simulink library "INT_CoTS_MechDem"  (R2016b)
settings: Solver=VariableStepAuto  StartTime=0.0  StopTime=10.0  RelTol=1e-3
settings Model: Creator=xinchangran  LastModifiedBy=xinchangran

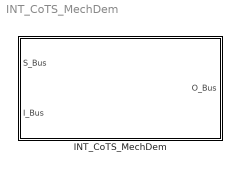
== system INT_CoTS_MechDem ==
  INT_CoTS_MechDem : Subsystem

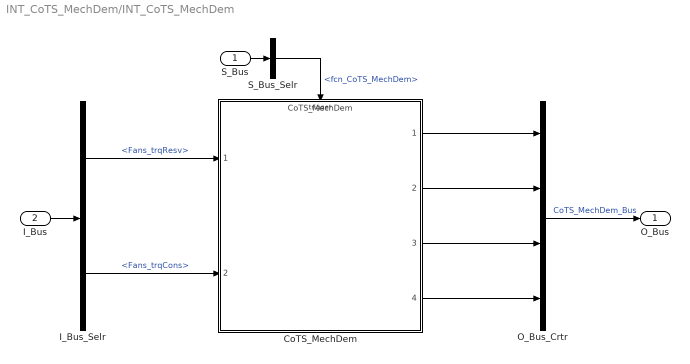
== system INT_CoTS_MechDem/INT_CoTS_MechDem ==
  S_Bus : Inport
  I_Bus : Inport  Port=2
  CoTS_MechDem : ModelReference  ModelNameDialog=CoTS_MechDem  SimulationMode=Normal  ModelReferenceVersion=1.19  TriggerPortName=function  TriggerPortTriggerType=function-call  TriggerPortStatesWhenEnabling=held
  I_Bus_Selr : BusSelector  OutputSignals=Fans_trqResv,Fans_trqCons
  O_Bus_Crtr : BusCreator  Inputs=4
  S_Bus_Selr : BusSelector  OutputSignals=fcn_CoTS_MechDem
  O_Bus : Outport
  wires:
  S_Bus_Selr/1 -> CoTS_MechDem/Trigger  "<fcn_CoTS_MechDem>"
  S_Bus/1 -> S_Bus_Selr/1
  I_Bus/1 -> I_Bus_Selr/1
  I_Bus_Selr/1 -> CoTS_MechDem/1  "<Fans_trqResv>"
  I_Bus_Selr/2 -> CoTS_MechDem/2  "<Fans_trqCons>"
  O_Bus_Crtr/1 -> O_Bus/1  "CoTS_MechDem_Bus"
  CoTS_MechDem/1 -> O_Bus_Crtr/1
  CoTS_MechDem/2 -> O_Bus_Crtr/2
  CoTS_MechDem/3 -> O_Bus_Crtr/3
  CoTS_MechDem/4 -> O_Bus_Crtr/4
